simulink library "sfun_storageTnodes"  (Simulink 8.2)
settings: Solver=ode45  StartTime=0.0  StopTime=10.0  RelTol=1e-3
settings Model: Creator=drhf  LastModifiedBy=drhf

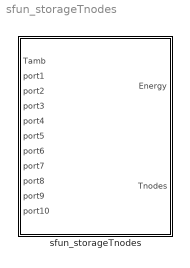
== system sfun_storageTnodes ==
  sfun_storageTnodes : Subsystem  mask(S-Function Storage T-Nodes){dia=0.5, volume=0.5, standing=1, uloss=1.1, ubot=1.1, utop=1.1, cond=0.9, tini=20, nodes=10, nconnect=10}
      mask prompts: dia "diameter [m]"; volume "volume [m³]"; standing "standing cylinder"; uloss "heat transfer coefficient to ambient [W/m²K]"; ubot "heat transfer coefficient to ambient bottom [W/m²K]"; utop "heat transfer coefficient to ambient top [W/m²K]"; cond "effective thermal conductivity [W/mK]"; tini "initial temperature [°C]"; nodes "number of nodes [1]"; nconnect "number of ports [1]"
      mask help:
      | Basic 1xN Model for a storage tank based on the equation. The flow is calculated by the upwind scheme heat conduction between nodes by central differences (Patankar 1980).
      | (rho*cp) * dT/dt =U * Aloss / Vnode * (Tamb - Tnode)
      | + cond / dh2 * (Tnode_above - Tnode)
      | + cond / dh2 * (Tnode_below - Tnode)
      | + mdot_up * cp / Vnode * (Tnode_below - Tnode)
      | + mdot_down * cp / Vnode * (Tnode_above - Tnode)
      | + Uhx * Ahx / Vnode * (Thx_node - Tnode)
      mask init:
      | if (floor(nodes)-nodes>eps(nodes)) || nodes < 1.0
      |     error('The number of nodes must be a positve integer!');
      | end
      | 
      | if (floor(nconnect)-nconnect>eps(nconnect)) || nconnect < 1.0
      |     error('The number of ports must be a positve integer!');
      | end
      | 
      | 
      | 
      | if numel(tini)==1
      |     tini = ones(int32(nodes), 1)*tini;
      | else
      |     if numel(tini)~=int32(nodes)
      |         error('The initialisation temperature must be a scalar or a vector of size of number of nodes!');
      |     end
      | end
      | 
      | CarnotCallbacks_storage_Tnodes('InitCallback', gcb, nconnect);
      mask Help: web(fullfile(path_carnot('help'),'sfun_storageTnodes.html'),'-helpbrowser')

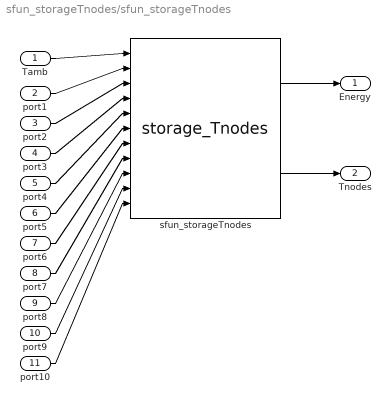
== system sfun_storageTnodes/sfun_storageTnodes ==
  Tamb : Inport
  port1 : Inport  Port=2
  port2 : Inport  Port=3
  port3 : Inport  Port=4
  port4 : Inport  Port=5
  port5 : Inport  Port=6
  port6 : Inport  Port=7
  port7 : Inport  Port=8
  port8 : Inport  Port=9
  port9 : Inport  Port=10
  port10 : Inport  Port=11
  sfun_storageTnodes : S-Function  FunctionName=storage_Tnodes  Parameters=dia, volume, standing, uloss , ubot, utop, cond, tini, nodes, nconnect  EnableBusSupport=off
  Energy : Outport
  Tnodes : Outport  Port=2
  wires:
  sfun_storageTnodes/1 -> Energy/1
  sfun_storageTnodes/2 -> Tnodes/1
  Tamb/1 -> sfun_storageTnodes/1
  port1/1 -> sfun_storageTnodes/2
  port2/1 -> sfun_storageTnodes/3
  port3/1 -> sfun_storageTnodes/4
  port4/1 -> sfun_storageTnodes/5
  port5/1 -> sfun_storageTnodes/6
  port6/1 -> sfun_storageTnodes/7
  port7/1 -> sfun_storageTnodes/8
  port8/1 -> sfun_storageTnodes/9
  port9/1 -> sfun_storageTnodes/10
  port10/1 -> sfun_storageTnodes/11
